simulink model "DAC"  (R2019a)
settings: Solver=VariableStepAuto  StartTime=0.0  StopTime=10.0  RelTol=1e-3
settings Model: Creator=chira  LastModifiedBy=Bhavya

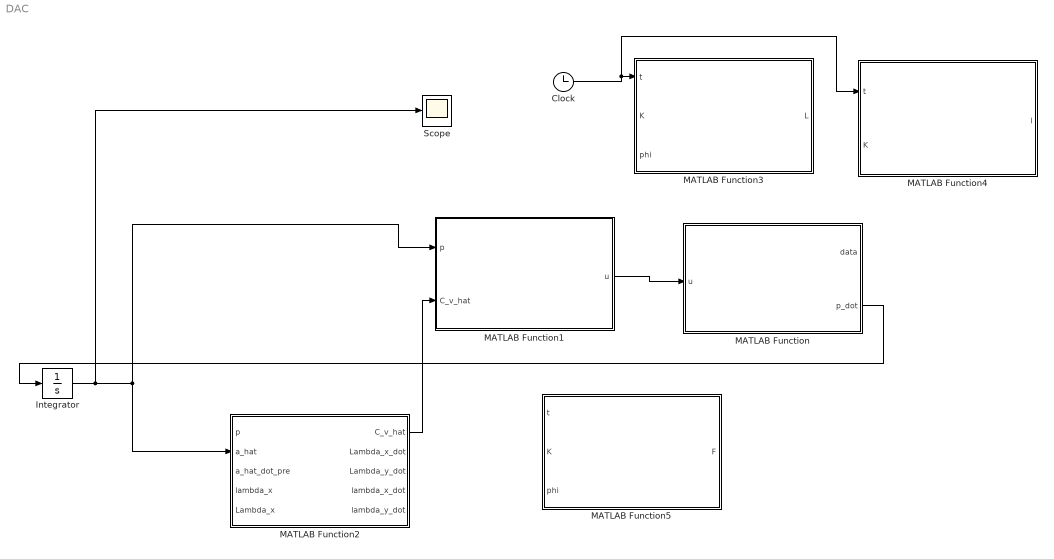
== system DAC ==
  Clock : Clock
  Integrator : Integrator
  MATLAB Function : MATLAB Function  TreatAsAtomicUnit=on
  MATLAB Function1 : MATLAB Function  TreatAsAtomicUnit=on
  MATLAB Function2 : MATLAB Function  TreatAsAtomicUnit=on
  MATLAB Function3 : MATLAB Function  TreatAsAtomicUnit=on
  MATLAB Function4 : MATLAB Function  TreatAsAtomicUnit=on
  MATLAB Function5 : MATLAB Function  TreatAsAtomicUnit=on
  Scope : Scope
  wires:
  MATLAB Function/2(p_dot) -> Integrator/1
  Integrator/1 -> Scope/1, MATLAB Function1/1(p), MATLAB Function2/2(a_hat)
  MATLAB Function2/1(C_v_hat) -> MATLAB Function1/2(C_v_hat)
  MATLAB Function1/1(u) -> MATLAB Function/1(u)
  Clock/1 -> MATLAB Function4/1(t), MATLAB Function3/1(t)

== matlab function DAC/MATLAB Function1 ==
  data: u output; p input; C_v_hat input
function u = controller(p,C_v_hat)
K=2*eye(2);
u=K*(C_v_hat-p);
end

== matlab function DAC/MATLAB Function ==
  data: data output; u input; p_dot output
function [data, p_dot] = dynamics(u)
p_dot=u;
end

== matlab function DAC/MATLAB Function2 ==
  data: p input; a_hat input; a_hat_dot_pre input; lambda_x input; C_v_hat output; Lambda_x_dot output; Lambda_y_dot output; lambda_x_dot output; Lambda_x input; lambda_y_dot output
function [C_v_hat,Lambda_x_dot,Lambda_y_dot,lambda_x_dot,lambda_y_dot]  = estimator(p,a_hat,a_hat_dot_pre,lambda_x,Lambda_x)
% mu=1;
% sigma=0.18;

if t==0
    a_hat=0.1;
    a_hat_dot_pre=0.1;
end
K=@(x) exp(-((x-1)'*(x-1)/(2*0.18.^2)));
phi=@(x) K(x)'*a_hat;
phix=@(x) x*phi(x);
% phi=@(y)gaussmf(y,[0.2,1]);

M_hat_x=integral(phi,0,1,'ArrayValued',true);
M_hat_y=integral(phi,0,1,'ArrayValued',true);
L_hat_x=integral(phix,0,1,'ArrayValued',true);
L_hat_y=integral(phix,0,1,'ArrayValued',true);
M_hat=M_hat_x*M_hat_y;
C_hat_x=L_hat_x/M_hat;
C_hat_y=L_hat_y/M_hat;
C_v_hat=[C_hat_x; C_hat_y];

Lambda_dot_fun=@(x) K(x)*K(x)';
lambda_dot_fun=@(x) K(x)*phi(x);

Lambda_x_dot=Lambda_dot_fun(p(0));
lambda_x_dot=lambda_dot_fun(p(0));
Lambda_y_dot=Lambda_dot_fun(p(1));
lambda_y_dot=lambda_dot_fun(p(1));

% Lambda_dot=[Lambda_x_dot;Lambda_y_dot];
% lambda_dot=[lambda_x_dot;lambda_y_dot];

F1_x_fun=@(x) K(x)*(x-p(0))';
F1_y_fun=@(y) K(y)*(y-p(1))';
F1xi=integral(F1_x_fun,0,1,'ArrayValued',true);
F1yi=integral(F1_y_fun,0,1,'ArrayValued',true);
F1=[F1xi,F1yi];
F2=[F1xi;F1yi];
F=F1*Kc*F2/M_hat;
tau=1.1;
if a_hat>0.1
    I=0;
elseif a_hat==0.1 && a_hat_dot_pre>=0
    I=0;
else
    I=1;
end
a_hat_dot=tau*(a_hat_dot_pre*(1-I));
end

== matlab function DAC/MATLAB Function3 ==
  data: L output; t input; K input; phi input
function L = Lambda(t,K,phi)
L=integrate(K*phi,0,t);
end

== matlab function DAC/MATLAB Function4 ==
  data: t input; K input; l output
function l = lam(t,K)
l=integrate(K*K,0,t);
end

== matlab function DAC/MATLAB Function5 ==
  data: F output; t input; K input; phi input
function F = Fi(t,K,phi)
Fn1=integral(K*,0,t);
end
